simulink model "RC_top_ACU"  (R2018b)
settings: Solver=VariableStepAuto  StartTime=0.0  StopTime=500000.0  RelTol=1e-3
libraries: simulink x4
(part 1 of 3)
settings Model: Creator=user  LastModifiedBy=user

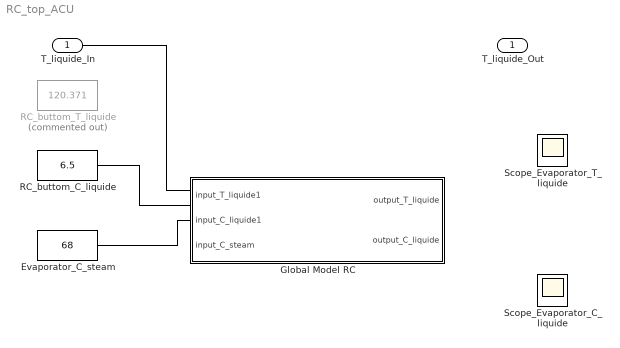
== system RC_top_ACU ==
  T_liquide_In : Inport
  Evaporator_C_steam : Constant  Value=68
  Global Model RC : Subsystem
  RC_buttom_C_liquide : Constant  Value=6.5
  RC_buttom_T_liquide : Constant  Commented=on  Value=120.371
  Scope_Evaporator_C_liquide : Scope
  Scope_Evaporator_T_liquide : Scope
  T_liquide_Out : Outport
  wires:
  ? -> T_liquide_Out/1, Scope_Evaporator_T_liquide/1
  ? -> Scope_Evaporator_C_liquide/1
  T_liquide_In/1 -> ?
  Evaporator_C_steam/1 -> ?
  RC_buttom_C_liquide/1 -> ?

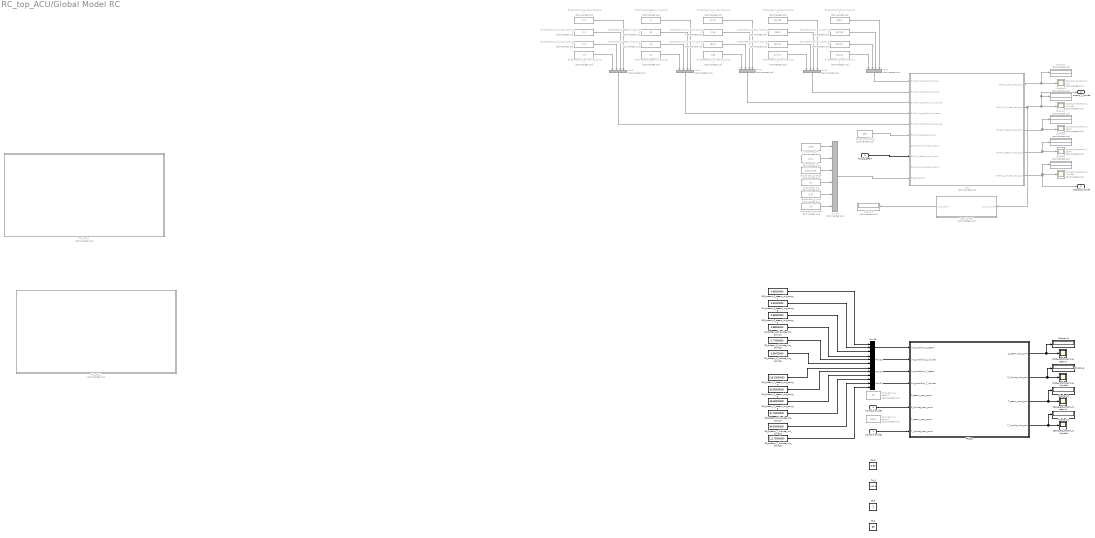
== system RC_top_ACU/Global Model RC ==
  input_T_liquide1 : Inport
  input_C_liquide1 : Inport  Port=2
  input_C_steam : Inport  Port=3
  ACU : Subsystem  Commented=on
  Cf_0 : Constant
  Cp_0 : Constant  Value=0.53
  Display{1..5,7} (6 alike) : Display  Commented=on
  Display{6,12..14} (4 alike) : Display
  Evaporator_C_liquide_init_point_1 : Constant  Commented=on  Value=2.2
  Evaporator_C_liquide_init_point_2 : Constant  Commented=on  Value=2.1
  Evaporator_C_liquide_init_point_3 : Constant  Commented=on  Value=2.0
  Evaporator_C_liquide_init_point_4 : Constant  Commented=on  Value=1.9
  Evaporator_C_steam_init_point_1 : Constant  Commented=on  Value=5
  Evaporator_C_steam_init_point_2 : Constant  Commented=on  Value=10
  Evaporator_C_steam_init_point_3 : Constant  Commented=on  Value=15
  Evaporator_C_steam_init_point_4 : Constant  Commented=on  Value=20
  Evaporator_Diameter : Constant  Commented=on  Value=5.5
  Evaporator_G_steam : Constant  Commented=on  Value=0.0017763
  Evaporator_P_0 : Constant  Commented=on  Value=0.1
  Evaporator_P_work : Constant  Commented=on  Value=0.06
  Evaporator_T_flue : Constant  Commented=on  Value=360
  Evaporator_T_flue_init_point_1 : Constant  Commented=on  Value=283.3
  Evaporator_T_flue_init_point_2 : Constant  Commented=on  Value=267.89
  Evaporator_T_flue_init_point_3 : Constant  Commented=on  Value=253.67
  Evaporator_T_flue_init_point_4 : Constant  Commented=on  Value=240.54
  Evaporator_T_liquide_init_point_1 : Constant  Commented=on  Value=137.5
  Evaporator_T_liquide_init_point_2 : Constant  Commented=on  Value=145
  Evaporator_T_liquide_init_point_3 : Constant  Commented=on  Value=152.5
  Evaporator_T_liquide_init_point_4 : Constant  Commented=on  Value=158
  Evaporator_T_side_init_point_1 : Constant  Commented=on  Value=164.48
  Evaporator_T_side_init_point_2 : Constant  Commented=on  Value=158.3
  Evaporator_T_side_init_point_3 : Constant  Commented=on  Value=152.41
  Evaporator_T_side_init_point_4 : Constant  Commented=on  Value=147.07
  Evaporator_Vm : Constant  Commented=on  Value=22.4
  Evaporator_dh : Constant  Commented=on  Value=1.375
  FULL_RC_1 : Subsystem  Commented=on
  FULL_RC_2 : Subsystem  Commented=on
  Local Control : Subsystem  Commented=on
  Mux10 : Mux  Commented=on  Inputs=6
  Mux{11..14} (4 alike) : Mux  Inputs=3
  Mux{5..9} (5 alike) : Mux  Commented=on
  RC_buttom_C_liquide_init_point_4 : Constant  Value=0.88825000
  RC_buttom_C_liquide_init_point_5 : Constant  Value=0.77650000
  RC_buttom_C_liquide_init_point_6 : Constant  Value=0.66475000
  RC_buttom_C_steam1 : Constant  Commented=on  Value=50
  RC_buttom_C_steam_init_point_4 : Constant  Value=0.68200000
  RC_buttom_C_steam_init_point_5 : Constant  Value=0.83400000
  RC_buttom_C_steam_init_point_6 : Constant  Value=0.98600000
  RC_buttom_T_liquide_init_point_4 : Constant  Value=57.25000000
  RC_buttom_T_liquide_init_point_5 : Constant  Value=84.50000000
  RC_buttom_T_liquide_init_point_6 : Constant  Value=111.75000000
  RC_buttom_T_steam1 : Constant  Commented=on  Value=150.4
  RC_buttom_T_steam_init_point_4 : Constant  Value=118.20000000
  RC_buttom_T_steam_init_point_5 : Constant  Value=93.90000000
  RC_buttom_T_steam_init_point_6 : Constant  Value=69.60000000
  RC_top : Subsystem
  Scope_Evaporator_C_liquide1 : Scope  Commented=on
  Scope_Evaporator_C_steam : Scope  Commented=on
  Scope_Evaporator_T_flue : Scope  Commented=on
  Scope_Evaporator_T_liquide1 : Scope  Commented=on
  Scope_Evaporator_T_steam : Scope  Commented=on
  Scope_RC_buttom_C_liquide1 : Scope
  Scope_RC_buttom_C_steam1 : Scope
  Scope_RC_buttom_T_liquide1 : Scope
  Scope_RC_buttom_T_steam1 : Scope
  Tf_0 : Constant  Value=30
  Tp_0 : Constant  Value=142.5
  output_T_liquide : Outport
  output_C_liquide : Outport  Port=2
  wires:
  RC_buttom_C_steam_init_point_6/1 -> Mux13/3
  RC_buttom_T_steam_init_point_6/1 -> Mux14/3
  RC_buttom_T_liquide_init_point_5/1 -> Mux12/2
  RC_buttom_C_steam_init_point_5/1 -> Mux13/2
  RC_buttom_C_liquide_init_point_5/1 -> Mux11/2
  RC_buttom_T_liquide_init_point_4/1 -> Mux12/1
  RC_top/1(C_steam_next_point) -> Display14/1, Scope_RC_buttom_C_steam1/1
  RC_buttom_C_liquide_init_point_4/1 -> Mux11/1
  Mux14/1 -> RC_top/3(init_condition_T_steam)
  input_C_liquide1/1 -> RC_top/6(C_liquide_prev_point)
  RC_top/2(C_liquide_next_point) -> Display6/1, Scope_RC_buttom_C_liquide1/1
  Mux12/1 -> RC_top/4(init_condition_T_liquide)
  RC_buttom_T_steam_init_point_5/1 -> Mux14/2
  Mux13/1 -> RC_top/1(init_condition_C_steam)
  input_T_liquide1/1 -> RC_top/8(T_liquide_prev_point)
  RC_buttom_T_liquide_init_point_6/1 -> Mux12/3
  RC_buttom_T_steam_init_point_4/1 -> Mux14/1
  RC_buttom_C_liquide_init_point_6/1 -> Mux11/3
  Mux11/1 -> RC_top/2(init_condition_C_liquide)
  RC_buttom_C_steam_init_point_4/1 -> Mux13/1
  RC_top/4(T_liquide_next_point) -> Display12/1, Scope_RC_buttom_T_liquide1/1
  RC_top/3(T_steam_next_point) -> Display13/1, Scope_RC_buttom_T_steam1/1
  Evaporator_T_liquide_init_point_3/1 -> Mux8/2
  Evaporator_T_side_init_point_4/1 -> Mux5/1
  Evaporator_T_side_init_point_2/1 -> Mux5/3
  Evaporator_C_steam_init_point_2/1 -> Mux6/3
  Evaporator_C_steam_init_point_3/1 -> Mux6/2
  Mux5/1 -> ACU/2(EVAP_init_condition_T_side)
  Evaporator_Vm/1 -> Mux10/2
  Mux7/1 -> ACU/1(EVAP_init_condition_T_flue)
  ACU/5(EVAP_C_liquide_next_point) -> Display7/1, Scope_Evaporator_C_liquide1/1, output_C_liquide/1
  ACU/1(EVAP_T_flue_next_point) -> Display2/1, Scope_Evaporator_T_flue/1
  Evaporator_C_steam_init_point_1/1 -> Mux6/4
  Evaporator_G_steam/1 -> Mux10/3
  Evaporator_T_liquide_init_point_1/1 -> Mux8/4
  ACU/4(EVAP_C_steam_next_point) -> Display4/1, Scope_Evaporator_C_steam/1
  Evaporator_C_liquide_init_point_3/1 -> Mux9/2
  Evaporator_P_work/1 -> Mux10/5
  Evaporator_T_flue_init_point_1/1 -> Mux7/4
  Evaporator_T_flue_init_point_4/1 -> Mux7/1
  Evaporator_T_liquide_init_point_4/1 -> Mux8/1
  Local Control/1(curr_T_flue) -> Display5/1
  Evaporator_C_liquide_init_point_2/1 -> Mux9/3
  Mux8/1 -> ACU/3(EVAP_init_condition_T_liquide)
  Evaporator_T_flue_init_point_2/1 -> Mux7/3
  Mux6/1 -> ACU/4(EVAP_init_condition_C_steam)
  Evaporator_P_0/1 -> Mux10/4
  Mux10/1 -> ACU/10(EVAP_params)
  Evaporator_T_flue_init_point_3/1 -> Mux7/2
  input_C_steam/1 -> ACU/8(EVAP_C_steam_prev_point)
  Evaporator_C_liquide_init_point_4/1 -> Mux9/1
  Evaporator_dh/1 -> Mux10/1
  Evaporator_T_side_init_point_3/1 -> Mux5/2
  ACU/3(EVAP_T_steam_next_point) -> Display1/1, Scope_Evaporator_T_steam/1
  Evaporator_Diameter/1 -> Mux10/6
  Mux9/1 -> ACU/5(EVAP_init_condition_C_liquide)
  Evaporator_C_steam_init_point_4/1 -> Mux6/1
  Evaporator_T_flue/1 -> ACU/6(EVAP_T_flue_prev_point)
  Evaporator_C_liquide_init_point_1/1 -> Mux9/4
  Evaporator_T_side_init_point_1/1 -> Mux5/4
  Evaporator_T_liquide_init_point_2/1 -> Mux8/3
  ACU/2(EVAP_T_liquide_next_point) -> output_T_liquide/1, Display3/1, Scope_Evaporator_T_liquide1/1, Local Control/1(curr_T_liquide)

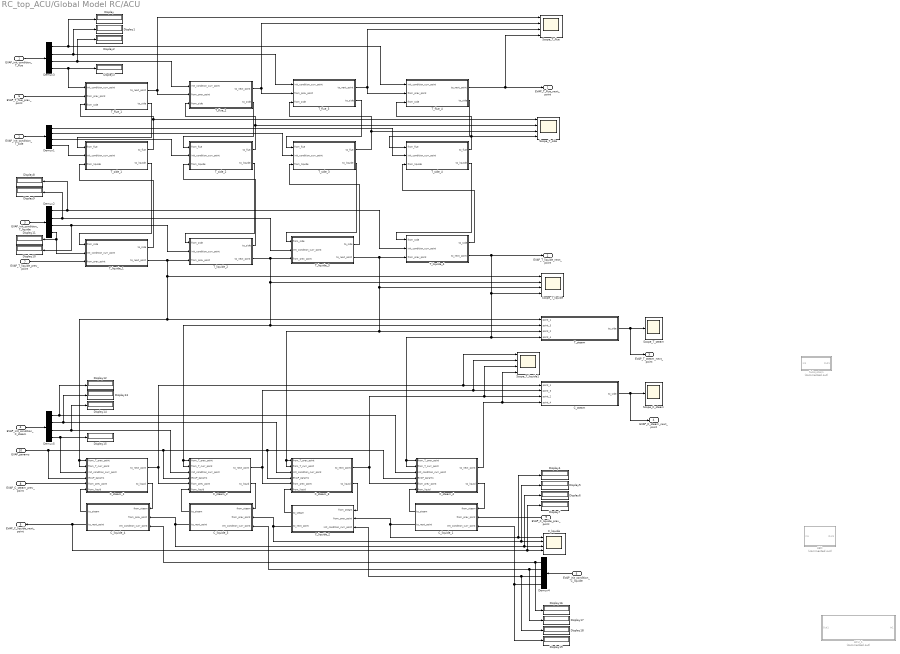
== system RC_top_ACU/Global Model RC/ACU ==
  EVAP_init_condition_T_flue : Inport
  EVAP_init_condition_T_side : Inport  Port=2
  EVAP_init_condition_T_liquide : Inport  Port=3
  EVAP_init_condition_C_steam : Inport  Port=4
  EVAP_init_condition_C_liquide : Inport  Port=5
  EVAP_T_flue_prev_point : Inport  Port=6
  EVAP_T_liquide_prev_point : Inport  Port=7
  EVAP_C_steam_prev_point : Inport  Port=8
  EVAP_C_liquide_prev_point : Inport  Port=9
  EVAP_params : Inport  Port=10
  "ACU_1 " : Subsystem  Commented=on
  C_liquide : Scope  NumInputPorts=4
  C_liquide_1 : Subsystem
  C_liquide_2 : Subsystem
  C_liquide_3 : Subsystem
  C_liquide_4 : Subsystem
  C_steam : Subsystem
  C_steam_1 : Subsystem
  C_steam_2 : Subsystem
  C_steam_3 : Subsystem
  C_steam_4 : Subsystem
  Demux{1..5} (5 alike) : Demux
  Display{,1..19} (20 alike) : Display
  Scope_C_steam : Scope
  Scope_T_flue : Scope  NumInputPorts=4
  Scope_T_liquide : Scope  NumInputPorts=4
  Scope_T_liquide1 : Scope  NumInputPorts=4
  Scope_T_side : Scope  NumInputPorts=4
  Scope_T_steam : Scope
  Subsystem : Subsystem  Commented=on
  T_flue_1 : Subsystem
  T_flue_2 : Subsystem
  T_flue_3 : Subsystem
  T_flue_4 : Subsystem
  T_liquide_1 : Subsystem
  T_liquide_2 : Subsystem
  T_liquide_3 : Subsystem
  T_liquide_4 : Subsystem
  T_side_1 : Subsystem
  T_side_2 : Subsystem
  T_side_3 : Subsystem
  T_side_4 : Subsystem
  T_steam : Subsystem
  АВО : Subsystem  Commented=on
  EVAP_T_flue_next_point : Outport
  EVAP_T_liquide_next_point : Outport  Port=2
  EVAP_T_steam_next_point : Outport  Port=3
  EVAP_C_steam_next_point : Outport  Port=4
  EVAP_C_liquide_next_point : Outport  Port=5
  wires:
  T_liquide_3/2(to_next_point) -> T_liquide_4/3(from_prev_point), C_steam_3/1(from_T_prev_point), C_steam_3/2(from_T_curr_point), T_steam/3(point_2), Scope_T_liquide/3
  EVAP_init_condition_T_liquide/1 -> Demux2/1
  Demux2/1 -> T_liquide_4/2(init_condition_curr_point), Display8/1
  EVAP_init_condition_T_side/1 -> Demux1/1
  T_liquide_4/2(to_next_point) -> Scope_T_liquide/4, C_steam_4/2(from_T_curr_point), C_steam_4/1(from_T_prev_point), T_steam/4(point_4), EVAP_T_liquide_next_point/1
  Demux2/2 -> T_liquide_3/2(init_condition_curr_point), Display9/1
  Demux2/4 -> T_liquide_1/2(init_condition_curr_point), Display11/1
  EVAP_init_condition_T_flue/1 -> Demux3/1
  T_flue_1/1(to_next_point) -> T_flue_2/2(from_prev_point), Scope_T_flue/1
  T_flue_2/1(to_next_point) -> T_flue_3/2(from_prev_point), Scope_T_flue/2
  T_flue_3/1(to_next_point) -> T_flue_4/2(from_prev_point), Scope_T_flue/3
  Demux3/1 -> T_flue_4/1(init_condition_curr_point), Display/1
  Demux3/2 -> T_flue_3/1(init_condition_curr_point), Display1/1
  Demux3/3 -> T_flue_2/1(init_condition_curr_point), Display2/1
  Demux3/4 -> T_flue_1/1(init_condition_curr_point), Display3/1
  T_flue_4/1(to_next_point) -> EVAP_T_flue_next_point/1, Scope_T_flue/4
  EVAP_T_flue_prev_point/1 -> T_flue_1/2(from_prev_point)
  T_steam/1(to_side) -> EVAP_T_steam_next_point/1, Scope_T_steam/1
  Demux5/2 -> C_steam_3/3(init_condition_curr_point), Display13/1
  C_liquide_2/2(to_next_point) -> C_liquide_3/2(from_prev_point), Display5/1, C_liquide/2
  C_steam_2/1(to_next_point) -> C_steam_3/5(from_prev_point), Scope_T_liquide1/2, C_steam/2(point_3)
  EVAP_init_condition_C_liquide/1 -> Demux4/1
  Demux5/3 -> C_steam_2/3(init_condition_curr_point), Display14/1
  C_steam_1/2(to_liquid) -> C_liquide_4/1(from_steam)
  Demux5/1 -> C_steam_4/3(init_condition_curr_point), Display12/1
  EVAP_init_condition_C_steam/1 -> Demux5/1
  EVAP_C_steam_prev_point/1 -> C_steam_1/5(from_prev_point)
  C_liquide_4/2(to_next_point) -> EVAP_C_liquide_next_point/1, Display7/1, C_liquide/4
  C_liquide_2/1(to_steam) -> C_steam_3/6(from_liquid)
  C_liquide_3/2(to_next_point) -> C_liquide_4/2(from_prev_point), Display6/1, C_liquide/3
  C_liquide_4/1(to_steam) -> C_steam_1/6(from_liquid)
  C_steam_3/1(to_next_point) -> C_steam_4/5(from_prev_point), Scope_T_liquide1/3, C_steam/3(point_2)
  EVAP_C_liquide_prev_point/1 -> C_liquide_1/2(from_prev_point)
  C_steam_4/2(to_liquid) -> C_liquide_1/1(from_steam)
  C_liquide_1/1(to_steam) -> C_steam_4/6(from_liquid)
  Demux5/4 -> C_steam_1/3(init_condition_curr_point), Display15/1
  C_liquide_1/2(to_next_point) -> C_liquide_2/2(from_prev_point), Display4/1, C_liquide/1
  Demux4/1 -> C_liquide_4/3(init_condition_curr_point), Display16/1
  Demux4/2 -> C_liquide_3/3(init_condition_curr_point), Display17/1
  Demux4/3 -> C_liquide_2/3(init_condition_curr_point), Display18/1
  Demux4/4 -> C_liquide_1/3(init_condition_curr_point), Display19/1
  C_steam/1(to_side) -> EVAP_C_steam_next_point/1, Scope_C_steam/1
  C_steam_1/1(to_next_point) -> C_steam_2/5(from_prev_point), Scope_T_liquide1/1, C_steam/1(point_1)
  C_steam_4/1(to_next_point) -> Scope_T_liquide1/4, C_steam/4(point_4)
  EVAP_params/1 -> C_steam_1/4(EVAP_params), C_steam_2/4(EVAP_params), C_steam_4/4(EVAP_params), C_steam_3/4(EVAP_params)
  C_liquide_3/1(to_steam) -> C_steam_2/6(from_liquid)
  C_steam_2/2(to_liquid) -> C_liquide_3/1(from_steam)
  EVAP_T_liquide_prev_point/1 -> T_liquide_1/3(from_prev_point)
  C_steam_3/2(to_liquid) -> C_liquide_2/1(from_steam)
  T_liquide_1/2(to_next_point) -> T_liquide_2/3(from_prev_point), Scope_T_liquide/1, T_steam/1(point_1), C_steam_1/1(from_T_prev_point), C_steam_1/2(from_T_curr_point)
  Demux2/3 -> T_liquide_2/2(init_condition_curr_point), Display10/1
  T_side_1/1(to_flue) -> Scope_T_side/1, T_flue_1/3(from_side)
  T_flue_1/2(to_side) -> T_side_1/1(from_flue)
  T_side_1/2(to_liquide) -> T_liquide_1/1(from_side)
  T_liquide_1/1(to_side) -> T_side_1/3(from_liquide)
  Demux1/4 -> T_side_1/2(init_condition_curr_point)
  T_side_2/1(to_flue) -> T_flue_2/3(from_side), Scope_T_side/2
  T_flue_2/2(to_side) -> T_side_2/1(from_flue)
  T_side_3/1(to_flue) -> T_flue_3/3(from_side), Scope_T_side/3
  T_flue_3/2(to_side) -> T_side_3/1(from_flue)
  T_side_4/1(to_flue) -> T_flue_4/3(from_side), Scope_T_side/4
  T_flue_4/2(to_side) -> T_side_4/1(from_flue)
  T_liquide_2/1(to_side) -> T_side_2/3(from_liquide)
  T_side_2/2(to_liquide) -> T_liquide_2/1(from_side)
  T_side_3/2(to_liquide) -> T_liquide_3/1(from_side)
  T_liquide_3/1(to_side) -> T_side_3/3(from_liquide)
  T_side_4/2(to_liquide) -> T_liquide_4/1(from_side)
  T_liquide_4/1(to_side) -> T_side_4/3(from_liquide)
  Demux1/3 -> T_side_2/2(init_condition_curr_point)
  Demux1/2 -> T_side_3/2(init_condition_curr_point)
  Demux1/1 -> T_side_4/2(init_condition_curr_point)
  T_liquide_2/2(to_next_point) -> T_liquide_3/3(from_prev_point), C_steam_2/2(from_T_curr_point), C_steam_2/1(from_T_prev_point), T_steam/2(point_3), Scope_T_liquide/2

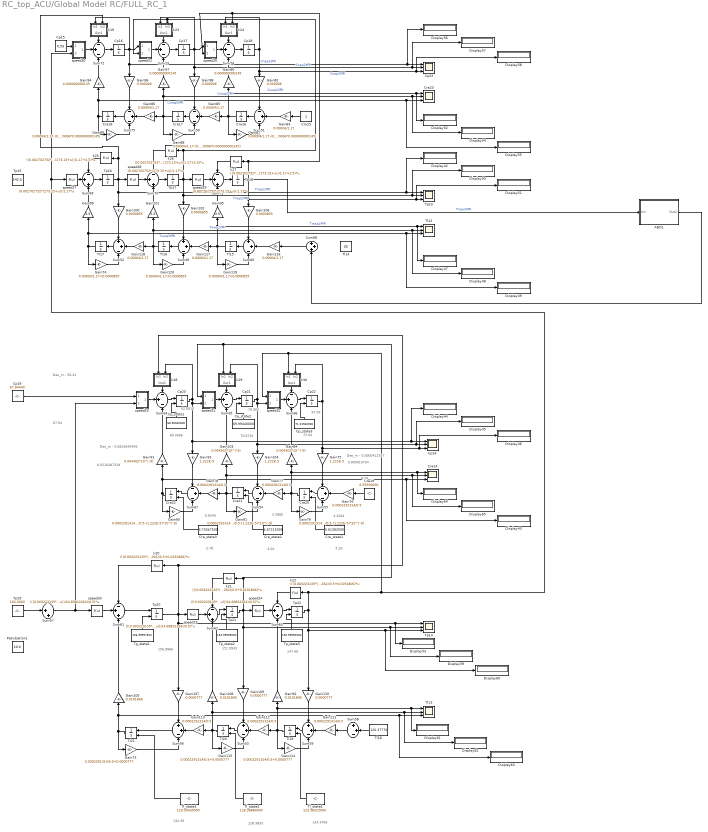
== system RC_top_ACU/Global Model RC/FULL_RC_1 ==
  note: 4.2264
  note: 69.3066
  note: 72.04
  note: 156.9966
  note: 124.3766
  note: 0.000010734
  note: 4.24
  note: Des_m - 0.0000412357
  note: 67.94
  note: Des_m - 50.41
  note: 4.02
  note: 147.99
  note: Des_m - 0.0815645409
  note: 0.0216487318
  note: 70.6733
  note: 2.3980
  note: 2.78
  note: 5.26
  note: 78.085
  note: 97.09
  note: 62.8910
  note: 0.9249
  note: 128.3833
  note: 151.9933
  note: 132.39
  Cp14 : Scope  NumInputPorts=3
  Cp15 : Constant  Value=0.53
  Cp16 : Integrator  InitialCondition=0.665
  Cp17 : Integrator  InitialCondition=0.803
  Cp18 : Integrator  InitialCondition=0.986
  Cp19 : Constant  Value=67.94440
  Cp20 : Integrator  InitialConditionSource=external  InitialCondition=69.3066
  Cp21 : Integrator  InitialConditionSource=external  InitialCondition=70.6733
  Cp22 : Integrator  InitialConditionSource=external  InitialCondition=72.04
  Cp23 : Scope  NumInputPorts=3
  Cp_state1 : Constant  Value=68.96940000
  Cp_state2 : Constant  Value=69.99440000
  Cp_state3 : Constant  Value=71.01940000
  Cra14 : Scope  NumInputPorts=3
  Cra15 : Constant
  Cra16 : Integrator  InitialCondition=0.827
  Cra17 : Integrator  InitialCondition=0.6862
  Cra18 : Integrator  InitialCondition=0.5696
  Cra19 : Constant  Value=6.55550000
  Cra20 : Integrator  InitialConditionSource=external  InitialCondition=5.26
  Cra21 : Integrator  InitialConditionSource=external  InitialCondition=4.02
  Cra22 : Integrator  InitialConditionSource=external  InitialCondition=2.78
  Cra23 : Scope  NumInputPorts=3
  Cra_state1 : Constant  Value=5.61382500
  Cra_state2 : Constant  Value=4.67215000
  Cra_state3 : Constant  Value=3.73047500
  Display{42..65} (24 alike) : Display
  Gain100 : Gain  Gain=0.0000855
  Gain101 : Gain  Gain=2.5
  Gain102 : Gain  Gain=0.0000855
  Gain103 : Gain  Gain=0.004302*10^(-9)
  Gain104 : Gain  Gain=1.222E-5
  Gain105 : Gain  Gain=0.0191806
  Gain106 : Gain  Gain=0.0000855
  Gain107 : Gain  Gain=0.0000777
  Gain108 : Gain  Gain=0.0191806
  Gain109 : Gain  Gain=0.0000777
  Gain110 : Gain  Gain=0.0000777
  Gain{76..78,111..113} (6 alike) : Gain  Gain=0.0002291314/0.5
  Gain114 : Gain  Gain=0.0002291314/0.5+0.0000777
  Gain115 : Gain  Gain=0.0002291314/0.5+0.0000777
  Gain{83,85..86,116..118} (6 alike) : Gain  Gain=0.00004/1.17
  Gain119 : Gain  Gain=0.00004/1.17+0.0000855
  Gain120 : Gain  Gain=0.00004/1.17+0.0000855
  Gain73 : Gain  Gain=0.0002291314/0.5+0.0000777
  Gain74 : Gain  Gain=0.00004/1.17+0.0000855
  Gain75 : Gain  Gain=1.222E-5
  Gain79 : Gain  Gain=0.0002291314/0.5-(1.222E-5)*10^(-9)
  Gain80 : Gain  Gain=0.000000000145
  Gain81 : Gain  Gain=0.0002291314/0.5-(1.222E-5)*10^(-9)
  Gain82 : Gain  Gain=0.000006
  Gain84 : Gain  Gain=0.004302*10^(-9)
  Gain87 : Gain  Gain=0.00004/1.17-(0.000006*0.000000000145)
  Gain88 : Gain  Gain=0.00004/1.17-(0.000006*0.000000000145)
  Gain89 : Gain  Gain=0.00004/1.17-(0.000006*0.000000000145)
  Gain90 : Gain  Gain=0.0002291314/0.5-(1.222E-5)*10^(-9)
  Gain91 : Gain  Gain=0.004302*10^(-9)
  Gain92 : Gain  Gain=0.0191806
  Gain93 : Gain  Gain=1.222E-5
  Gain94 : Gain  Gain=0.000000000145
  Gain95 : Gain  Gain=2.5
  Gain96 : Gain  Gain=0.000006
  Gain97 : Gain  Gain=0.000000000145
  Gain98 : Gain  Gain=0.000006
  Gain99 : Gain  Gain=2.5
  Petrubation1 : Constant  Value=10.0
  Sum{49,52..53,56,58..60} (7 alike) : Sum  Inputs=++-
  Sum{50..51,54..55,64..67,72..75} (12 alike) : Sum  Inputs=-+-
  Sum57 : Sum  Inputs=|++
  Sum{61..63,69..71} (6 alike) : Sum  Inputs=-++
  Sum68 : Sum  Inputs=+++
  Tl13 : Scope  NumInputPorts=3
  Tl14 : Constant  Value=30
  Tl15 : Integrator  InitialCondition=58.28
  Tl16 : Integrator  InitialCondition=86.23
  Tl17 : Integrator  InitialCondition=111.75
  Tl18 : Constant  Value=120.37770
  Tl19 : Integrator  InitialConditionSource=external  InitialCondition=124.3766
  Tl20 : Integrator  InitialConditionSource=external  InitialCondition=128.3833
  Tl21 : Integrator  InitialConditionSource=external  InitialCondition=132.39
  Tl22 : Scope  NumInputPorts=3
  "Tl_state1 " : Constant  Value=123.38325000
  Tl_state2 : Constant  Value=126.38880000
  Tl_state3 : Constant  Value=129.39435000
  Tp14 : Scope  NumInputPorts=3
  Tp15 : Constant  Value=142.5
  Tp16 : Integrator  InitialCondition=121.956
  Tp17 : Integrator  InitialCondition=97.4
  Tp18 : Integrator  InitialCondition=69.6  IgnoreLimit=on
  Tp19 : Constant  Value=160.0000
  Tp20 : Integrator  InitialConditionSource=external  InitialCondition=156.9966
  Tp21 : Integrator  InitialConditionSource=external  InitialCondition=151.9933
  Tp22 : Integrator  InitialConditionSource=external  InitialCondition=147.99  IgnoreLimit=on
  Tp23 : Scope  NumInputPorts=3
  Tp_state1 : Constant  Value=156.99997500
  Tp_state2 : Constant  Value=153.99995000
  Tp_state3 : Constant  Value=150.99992500
  k19 : Subsystem
  k20 : Fcn  Expr=(((0.003223135*(273+u))/24.69822264)/0.5+0.0191806)*u
  k21 : Fcn  Expr=(((0.003223135*(273+u))/24.69822264)/0.5+0.0191806)*u
  k22 : Fcn  Expr=(((0.003223135*(273+u))/24.69822264)/0.5+0.0191806)*u
  k23 : Subsystem
  k24 : Subsystem
  k25 : Fcn  Expr=((0.002702752*(273.15+u))/1.17+2.5)*u
  k26 : Fcn  Expr=((0.002702752*(273.15+u))/1.17+2.5)*u
  k27 : Fcn  Expr=((0.002702752*(273.15+u))/1.17+2.5)*u
  k28 : Subsystem
  k29 : Subsystem
  k30 : Subsystem
  speed22 : Subsystem
  speed23 : Fcn  Expr=(((0.003223135*(273+u))/24.69822264)/0.5)*u
  speed24 : Fcn  Expr=(((0.003223135*(273+u))/24.69822264)/0.5)*u
  speed25 : Subsystem
  speed26 : Subsystem
  speed27 : Fcn  Expr=(0.002702752*(273.15+u))/1.17*u
  speed28 : Fcn  Expr=(0.002702752*(273.15+u))/1.17*u
  speed29 : Fcn  Expr=(0.002702752*(273.15+u))/1.17*u
  speed30 : Subsystem
  speed31 : Subsystem
  speed32 : Subsystem
  speed33 : Fcn  Expr=(((0.003223135*(273+u))/24.69822264)/0.5)*u
  АВО1 : Subsystem
  wires:
  k30/1(Out1) -> Sum66/1
  Tl19/1 -> Gain114/1, Gain112/1, Gain92/1, Display61/1, Tl13/1
  speed25/1(Out1) -> Sum64/2
  Tp_state1/1 -> Tp20/2
  Gain109/1 -> Sum53/1
  Gain113/1 -> Sum56/2
  speed22/1(Out1) -> Sum73/2
  Cp20/1 -> speed31/2(In2), Gain93/1, Cp14/1, Display44/1, k28/2(In2)
  Tl21/1 -> Gain73/1, Gain105/1, Display63/1, Tl13/3
  Cp15/1 -> speed30/1(In1)
  Sum63/1 -> Tp22/1
  Cp16/1 -> Cp23/1, Display56/1, Gain96/1, k19/1(In1), speed22/1(In1)  "Cпар1УРК"
  Tp16/1 -> Display42/1, Tp23/1, Gain100/1, k25/1, k19/2(In2), speed28/1  "Tпар1УРК"
  speed26/1(Out1) -> Sum74/2
  Gain89/1 -> Sum75/3
  speed27/1 -> Sum69/2
  Sum49/1 -> Tl16/1
  Sum56/1 -> Tl21/1
  k27/1 -> Sum71/1
  Gain116/1 -> Sum60/2
  Gain81/1 -> Sum54/3
  k26/1 -> Sum70/1
  speed31/1(Out1) -> Sum65/2
  Gain99/1 -> Sum69/3
  Gain94/1 -> Sum72/3
  Sum73/1 -> Cp17/1
  Gain82/1 -> Sum51/1
  Sum74/1 -> Cp18/1
  Sum69/1 -> Tp16/1
  Cra19/1 -> Gain76/1
  k20/1 -> Sum61/1
  Gain97/1 -> Sum73/3
  Tp18/1 -> АВО1/1(In1), Display51/1, Tp23/3, Gain106/1, k27/1, k24/2(In2), speed26/2(In2)  "Tпар3УРК"
  Gain91/1 -> Sum64/3
  speed23/1 -> Sum62/2
  Gain80/1 -> Sum74/3
  "Tl_state1 "/1 -> Tl19/2
  Tp20/1 -> Gain107/1, Display53/1, Tp14/1, k20/1, k28/1(In1), speed23/1
  Gain95/1 -> Sum71/3
  Sum50/1 -> Cra17/1
  Gain98/1 -> Sum50/1
  k19/1(Out1) -> Sum72/1
  Gain106/1 -> Sum60/1
  Tp21/1 -> Gain109/1, Display59/1, Tp14/2, k21/1, speed31/1(In1), k29/1(In1), speed24/1
  Tp_state3/1 -> Tp22/2
  k21/1 -> Sum62/1
  Sum75/1 -> Cra18/1
  speed30/1(Out1) -> Sum72/2
  Sum72/1 -> Cp16/1
  Sum52/1 -> Tl17/1
  Cp_state3/1 -> Cp22/2
  Gain120/1 -> Sum49/3
  Gain79/1 -> Sum55/3
  Sum70/1 -> Tp17/1
  Tl15/1 -> Gain119/1, Gain117/1, Display47/1, Tl22/1, Gain95/1  "Tжид1УРК"
  Gain85/1 -> Sum50/2
  Tl18/1 -> Sum58/2
  Cp17/1 -> Display57/1, Cp23/2, Gain98/1, speed26/1(In1), k23/1(In1)  "Cпар2УРК"
  Tl_state3/1 -> Tl21/2
  Gain100/1 -> Sum52/1
  Tl16/1 -> Gain120/1, Gain118/1, Display48/1, Tl22/2, Gain101/1  "Tжид2УРК"
  Cra17/1 -> Gain88/1, Gain86/1, Display54/1, Cra23/2, Gain97/1  "Cжид2УРК"
  Gain104/1 -> Sum54/1
  Sum57/1 -> speed33/1, speed25/2(In2)
  Gain78/1 -> Sum67/2
  Cp22/1 -> k30/2(In2), Gain75/1, Display46/1, Cp14/3
  Gain84/1 -> Sum66/3
  Gain117/1 -> Sum49/2
  Sum65/1 -> Cp21/1
  Gain118/1 -> Sum52/2
  Gain87/1 -> Sum51/3
  Cra20/1 -> Gain79/1, Gain77/1, Gain84/1, Display64/1, Cra14/1
  Sum61/1 -> Tp20/1
  Sum62/1 -> Tp21/1
  Gain101/1 -> Sum70/3
  Gain86/1 -> Sum75/2
  Sum67/1 -> Cra22/1
  Gain75/1 -> Sum55/1
  speed28/1 -> Sum70/2
  Sum66/1 -> Cp22/1
  Sum58/1 -> Gain111/1
  Sum71/1 -> Tp18/1
  Gain111/1 -> Sum59/2
  speed29/1 -> Sum71/2
  Cra18/1 -> Gain89/1, Display55/1, Cra23/3, Gain94/1  "Cжид3УРК"
  k23/1(Out1) -> Sum73/1
  Gain110/1 -> Sum59/1
  Gain83/1 -> Sum51/2
  Sum55/1 -> Cra20/1
  k24/1(Out1) -> Sum74/1
  Gain119/1 -> Sum60/3
  Cra16/1 -> Gain87/1, Gain85/1, Display52/1, Cra23/1, Gain80/1  "Cжид1УРК"
  Gain114/1 -> Sum59/3
  Sum51/1 -> Cra16/1
  Gain90/1 -> Sum67/3
  k28/1(Out1) -> Sum64/1
  Gain88/1 -> Sum50/3
  Tl20/1 -> Gain115/1, Gain113/1, Gain108/1, Display62/1, Tl13/2
  Cra_state1/1 -> Cra20/2
  Tp22/1 -> Gain110/1, Display60/1, Tp14/3, k22/1, k30/1(In1), speed32/1(In1), speed30/2(In2), speed27/1
  Gain92/1 -> Sum63/3
  Cp_state2/1 -> Cp21/2
  Tp19/1 -> Sum57/1
  k25/1 -> Sum69/1
  Sum59/1 -> Tl19/1
  k22/1 -> Sum63/1
  speed24/1 -> Sum63/2
  Cp_state1/1 -> Cp20/2
  Gain105/1 -> Sum61/3
  Gain77/1 -> Sum54/2
  speed33/1 -> Sum61/2
  Gain112/1 -> Sum53/2
  k29/1(Out1) -> Sum65/1
  Cra15/1 -> Gain83/1
  Tp_state2/1 -> Tp21/2
  Gain93/1 -> Sum67/1
  Gain74/1 -> Sum52/3
  Tp17/1 -> Display50/1, Tp23/2, Gain102/1, k26/1, speed22/2(In2), k23/2(In2), speed29/1  "Tпар2УРК"
  Cra22/1 -> Gain90/1, Gain91/1, Display43/1, Cra14/3
  Sum64/1 -> Cp20/1
  Cra_state2/1 -> Cra21/2
  Cp19/1 -> speed25/1(In1)
  АВО1/1(Out1) -> Sum68/3
  Sum53/1 -> Tl20/1
  Gain115/1 -> Sum53/3
  Gain73/1 -> Sum56/3
  Tl_state2/1 -> Tl20/2
  Sum60/1 -> Tl15/1
  Gain76/1 -> Sum55/2
  Gain103/1 -> Sum65/3
  Cp21/1 -> speed32/2(In2), Gain104/1, Display45/1, Cp14/2, k29/2(In2)
  Cra_state3/1 -> Cra22/2
  Sum54/1 -> Cra21/1
  Gain96/1 -> Sum75/1
  Gain102/1 -> Sum49/1
  Cp18/1 -> Display58/1, Cp23/3, Gain82/1, k24/1(In1)  "Cпар3УРК"
  Gain108/1 -> Sum62/3
  Gain107/1 -> Sum56/1
  Cra21/1 -> Gain81/1, Gain78/1, Gain103/1, Display65/1, Cra14/2
  speed32/1(Out1) -> Sum66/2
  Tl17/1 -> Gain74/1, Display49/1, Tl22/3, Gain99/1  "Tжид3УРК"
  Sum68/1 -> Gain116/1

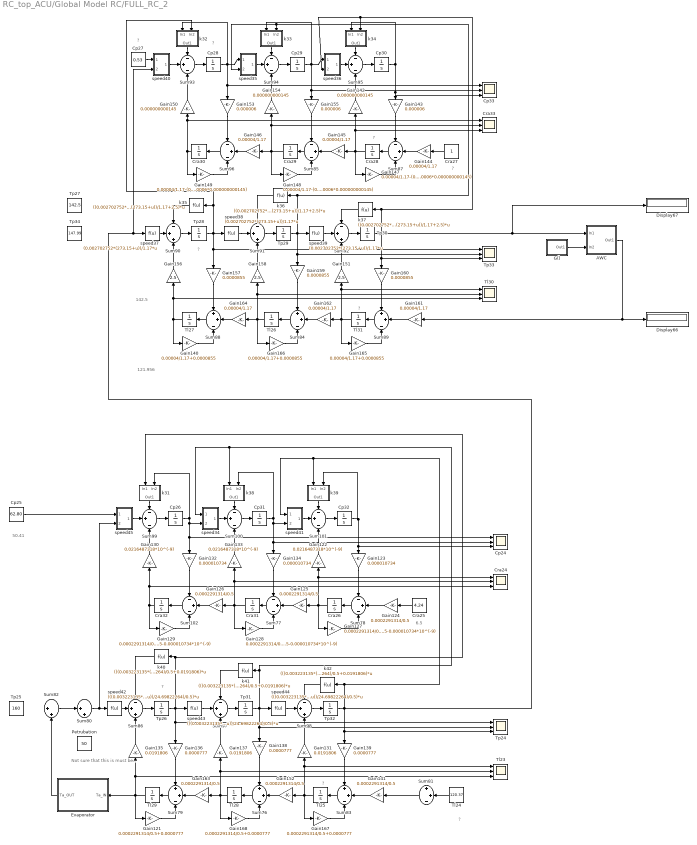
== system RC_top_ACU/Global Model RC/FULL_RC_2 ==
  note: ?
  note: Not sure that
      | this is must be..
  note: ?
  note: ?
  note: 142.5
  note: 50.41
  note: 6.5
  note: ?
  note: ?
  note: ?
  note: ?
  note: 121.956
  note: ?
  note: ?
  AWC : Subsystem
  Cp24 : Scope  NumInputPorts=3
  Cp25 : Constant  Value=62.80
  Cp26 : Integrator  InitialCondition=62.80
  Cp27 : Constant  Value=0.53
  Cp28 : Integrator  InitialCondition=0.665
  Cp29 : Integrator  InitialCondition=0.803
  Cp30 : Integrator  InitialCondition=0.986
  Cp31 : Integrator  InitialCondition=77.79
  Cp32 : Integrator  InitialCondition=96.56
  Cp33 : Scope  NumInputPorts=3
  Cra24 : Scope  NumInputPorts=3
  Cra25 : Constant  Value=4.24
  Cra26 : Integrator  InitialCondition=4.24
  Cra27 : Constant
  Cra28 : Integrator  InitialCondition=0.827
  Cra29 : Integrator  InitialCondition=0.6862
  Cra30 : Integrator  InitialCondition=0.5696
  Cra31 : Integrator  InitialCondition=2.42
  Cra32 : Integrator  InitialCondition=0.95
  Cra33 : Scope  NumInputPorts=3
  Display66 : Display
  Display67 : Display
  Evaporator : Subsystem
  G() : Subsystem
  Gain121 : Gain  Gain=0.0002291314/0.5+0.0000777
  Gain122 : Gain  Gain=0.0216487318*10^(-9)
  Gain123 : Gain  Gain=0.000010734
  Gain{124..126,141,152,163} (6 alike) : Gain  Gain=0.0002291314/0.5
  Gain127 : Gain  Gain=0.0002291314/0.5-0.000010734*10^(-9)
  Gain128 : Gain  Gain=0.0002291314/0.5-0.000010734*10^(-9)
  Gain129 : Gain  Gain=0.0002291314/0.5-0.000010734*10^(-9)
  Gain130 : Gain  Gain=0.0216487318*10^(-9)
  Gain131 : Gain  Gain=0.0191806
  Gain132 : Gain  Gain=0.000010734
  Gain133 : Gain  Gain=0.0216487318*10^(-9)
  Gain134 : Gain  Gain=0.000010734
  Gain135 : Gain  Gain=0.0191806
  Gain136 : Gain  Gain=0.0000777
  Gain137 : Gain  Gain=0.0191806
  Gain138 : Gain  Gain=0.0000777
  Gain139 : Gain  Gain=0.0000777
  Gain140 : Gain  Gain=0.00004/1.17+0.0000855
  Gain142 : Gain  Gain=0.000000000145
  Gain143 : Gain  Gain=0.000006
  Gain{144..146,161..162,164} (6 alike) : Gain  Gain=0.00004/1.17
  Gain147 : Gain  Gain=0.00004/1.17-(0.000006*0.000000000145)
  Gain148 : Gain  Gain=0.00004/1.17-(0.000006*0.000000000145)
  Gain149 : Gain  Gain=0.00004/1.17-(0.000006*0.000000000145)
  Gain150 : Gain  Gain=0.000000000145
  Gain151 : Gain  Gain=2.5
  Gain153 : Gain  Gain=0.000006
  Gain154 : Gain  Gain=0.000000000145
  Gain155 : Gain  Gain=0.000006
  Gain156 : Gain  Gain=2.5
  Gain157 : Gain  Gain=0.0000855
  Gain158 : Gain  Gain=2.5
  Gain159 : Gain  Gain=0.0000855
  Gain160 : Gain  Gain=0.0000855
  Gain165 : Gain  Gain=0.00004/1.17+0.0000855
  Gain166 : Gain  Gain=0.00004/1.17+0.0000855
  Gain167 : Gain  Gain=0.0002291314/0.5+0.0000777
  Gain168 : Gain  Gain=0.0002291314/0.5+0.0000777
  Petrubation : Constant  Value=50
  Sum{77..78,85,87,93..96,99..102} (12 alike) : Sum  Inputs=-+-
  Sum{76,79,81,83..84,88..89} (7 alike) : Sum  Inputs=++-
  Sum80 : Sum  Inputs=|++
  Sum82 : Sum  Inputs=|++
  Sum{86,90..92,97..98} (6 alike) : Sum  Inputs=-++
  Tl23 : Scope  NumInputPorts=3
  Tl24 : Constant  Value=120.37
  Tl25 : Integrator  InitialCondition=120.37
  Tl26 : Integrator  InitialCondition=86.23
  Tl27 : Integrator  InitialCondition=111.75
  Tl28 : Integrator  InitialCondition=124.37
  Tl29 : Integrator  InitialCondition=128.38
  Tl30 : Scope  NumInputPorts=3
  Tl31 : Integrator  InitialCondition=58.28
  Tp24 : Scope  NumInputPorts=3
  Tp25 : Constant  Value=160
  Tp26 : Integrator  InitialCondition=160
  Tp27 : Constant  Value=142.5
  Tp28 : Integrator  InitialCondition=121.956
  Tp29 : Integrator  InitialCondition=97.4
  Tp30 : Integrator  InitialCondition=69.6  IgnoreLimit=on
  Tp31 : Integrator  InitialCondition=157.34
  Tp32 : Integrator  InitialCondition=153.75  IgnoreLimit=on
  Tp33 : Scope  NumInputPorts=3
  Tp34 : Constant  Value=147.99
  k31 : Subsystem
  k32 : Subsystem
  k33 : Subsystem
  k34 : Subsystem
  k35 : Fcn  Expr=((0.002702752*(273.15+u))/1.17+2.5)*u
  k36 : Fcn  Expr=((0.002702752*(273.15+u))/1.17+2.5)*u
  k37 : Fcn  Expr=((0.002702752*(273.15+u))/1.17+2.5)*u
  k38 : Subsystem
  k39 : Subsystem
  k40 : Fcn  Expr=(((0.003223135*(273+u))/24.69822264)/0.5+0.0191806)*u
  k41 : Fcn  Expr=(((0.003223135*(273+u))/24.69822264)/0.5+0.0191806)*u
  k42 : Fcn  Expr=(((0.003223135*(273+u))/24.69822264)/0.5+0.0191806)*u
  speed34 : Subsystem
  speed35 : Subsystem
  speed36 : Subsystem
  speed37 : Fcn  Expr=(0.002702752*(273.15+u))/1.17*u
  speed38 : Fcn  Expr=(0.002702752*(273.15+u))/1.17*u
  speed39 : Fcn  Expr=(0.002702752*(273.15+u))/1.17*u
  speed40 : Subsystem
  speed41 : Subsystem
  speed42 : Fcn  Expr=(((0.003223135*(273+u))/24.69822264)/0.5)*u
  speed43 : Fcn  Expr=(((0.003223135*(273+u))/24.69822264)/0.5)*u
  speed44 : Fcn  Expr=(((0.003223135*(273+u))/24.69822264)/0.5)*u
  speed45 : Subsystem
  wires:
  Gain144/1 -> Sum87/2
  Sum85/1 -> Cra29/1
  Cra28/1 -> Gain147/1, Gain145/1, Cra33/3, Gain142/1
  Gain153/1 -> Sum96/1
  Cra30/1 -> Gain149/1, Cra33/1, Gain150/1
  Cp28/1 -> Cp33/1, Gain153/1, speed35/1(In1), k32/1(In1)
  Cra25/1 -> Gain124/1
  Cra31/1 -> Gain128/1, Gain126/1, Gain133/1, Cra24/2
  Cp32/1 -> k39/2(In2), Gain123/1, Cp24/3
  speed39/1 -> Sum92/2
  Gain146/1 -> Sum96/2
  k35/1 -> Sum90/1
  Sum97/1 -> Tp31/1
  Gain123/1 -> Sum78/1
  speed43/1 -> Sum97/2
  Sum96/1 -> Cra30/1
  Gain142/1 -> Sum95/3
  Tp32/1 -> Gain139/1, Tp24/3, speed40/2(In2), speed37/1, k42/1, k39/1(In1), speed41/1(In1)
  Tp31/1 -> Gain138/1, Tp24/2, k41/1, speed34/1(In1), k38/1(In1), speed44/1
  Cra27/1 -> Gain144/1
  Tp28/1 -> Gain157/1, Tp33/1, k35/1, k32/2(In2), speed38/1
  Sum81/1 -> Gain141/1
  Gain156/1 -> Sum90/3
  Gain151/1 -> Sum92/3
  Gain162/1 -> Sum84/2
  Gain155/1 -> Sum85/1
  Sum91/1 -> Tp29/1
  Tp29/1 -> Gain159/1, Tp33/2, k36/1, speed35/2(In2), k33/2(In2), speed39/1
  Tl31/1 -> Gain165/1, Gain162/1, Tl30/1, Gain151/1
  speed38/1 -> Sum91/2
  Cra32/1 -> Gain129/1, Gain130/1, Cra24/3
  Sum98/1 -> Tp32/1
  Gain163/1 -> Sum79/2
  Tl25/1 -> Gain167/1, Gain152/1, Gain131/1, Tl23/1
  k31/1(Out1) -> Sum99/1
  Sum78/1 -> Cra26/1
  speed41/1(Out1) -> Sum101/2
  Gain167/1 -> Sum83/3
  Gain150/1 -> Sum93/3
  Gain158/1 -> Sum91/3
  Cp29/1 -> Cp33/2, Gain155/1, speed36/1(In1), k33/1(In1)
  Sum94/1 -> Cp29/1
  k38/1(Out1) -> Sum100/1
  k40/1 -> Sum86/1
  Tl28/1 -> Gain168/1, Gain163/1, Gain137/1, Tl23/2
  Sum92/1 -> Tp30/1
  Gain154/1 -> Sum94/3
  Sum84/1 -> Tl26/1
  Gain121/1 -> Sum79/3
  k41/1 -> Sum97/1
  speed35/1(Out1) -> Sum94/2
  Gain131/1 -> Sum98/3
  Gain138/1 -> Sum76/1
  Gain141/1 -> Sum83/2
  Sum90/1 -> Tp28/1
  Gain157/1 -> Sum88/1
  Gain159/1 -> Sum84/1
  Gain136/1 -> Sum79/1
  Sum82/1 -> Sum80/1
  Gain128/1 -> Sum77/3
  Gain140/1 -> Sum88/3
  speed37/1 -> Sum90/2
  Sum99/1 -> Cp26/1
  k42/1 -> Sum98/1
  Sum80/1 -> speed45/2(In2), speed42/1
  Tp26/1 -> Gain136/1, Tp24/1, k40/1, k31/1(In1), speed43/1
  Sum89/1 -> Tl31/1
  Gain149/1 -> Sum96/3
  Gain148/1 -> Sum85/3
  k34/1(Out1) -> Sum95/1
  Cra29/1 -> Gain148/1, Gain146/1, Cra33/2, Gain154/1
  Tp30/1 -> AWC/1(In1), Display67/1, Gain160/1, Tp33/3, k37/1, k34/2(In2), speed36/2(In2)
  Sum93/1 -> Cp28/1
  Gain134/1 -> Sum77/1
  Gain127/1 -> Sum78/3
  Gain129/1 -> Sum102/3
  Gain161/1 -> Sum89/2
  speed42/1 -> Sum86/2
  Sum86/1 -> Tp26/1
  Cp26/1 -> speed34/2(In2), Gain132/1, Cp24/1, k31/2(In2)
  speed36/1(Out1) -> Sum95/2
  AWC/1(Out1) -> Display66/1, Gain161/1
  speed44/1 -> Sum98/2
  Sum102/1 -> Cra32/1
  Gain124/1 -> Sum78/2
  speed45/1(Out1) -> Sum99/2
  Sum77/1 -> Cra31/1
  Sum76/1 -> Tl28/1
  Tl26/1 -> Gain166/1, Gain164/1, Tl30/2, Gain158/1
  Gain135/1 -> Sum86/3
  Sum87/1 -> Cra28/1
  k36/1 -> Sum91/1
  speed34/1(Out1) -> Sum100/2
  Gain122/1 -> Sum101/3
  Evaporator/1(Ta_OUT) -> Sum82/2
  Sum88/1 -> Tl27/1
  speed40/1(Out1) -> Sum93/2
  Gain166/1 -> Sum84/3
  Gain145/1 -> Sum85/2
  Gain147/1 -> Sum87/3
  Gain152/1 -> Sum76/2
  Gain165/1 -> Sum89/3
  Cp25/1 -> speed45/1(In1)
  Cra26/1 -> Gain127/1, Gain125/1, Gain122/1, Cra24/1
  Gain143/1 -> Sum87/1
  Cp27/1 -> speed40/1(In1)
  Gain125/1 -> Sum77/2
  Gain168/1 -> Sum76/3
  Tl24/1 -> Sum81/2
  k37/1 -> Sum92/1
  Gain164/1 -> Sum88/2
  Sum79/1 -> Tl29/1
  k33/1(Out1) -> Sum94/1
  Gain130/1 -> Sum99/3
  Gain132/1 -> Sum102/1
  Gain126/1 -> Sum102/2
  Sum101/1 -> Cp32/1
  Cp31/1 -> speed41/2(In2), Gain134/1, Cp24/2, k38/2(In2)
  Cp30/1 -> Cp33/3, Gain143/1, k34/1(In1)
  Gain137/1 -> Sum97/3
  Tl29/1 -> Evaporator/1(Ta_IN), Gain121/1, Gain135/1, Tl23/3
  Gain133/1 -> Sum100/3
  k32/1(Out1) -> Sum93/1
  Gain160/1 -> Sum89/1
  Sum83/1 -> Tl25/1
  Gain139/1 -> Sum83/1
  k39/1(Out1) -> Sum101/1
  G()/1(Out1) -> AWC/2(In2)
  Tl27/1 -> Gain140/1, Gain156/1, Tl30/3
  Sum100/1 -> Cp31/1
  Sum95/1 -> Cp30/1

== system RC_top_ACU/Global Model RC/Local Control ==
  curr_T_liquide : Inport
  %/c : RateLimiter  RisingSlewLimit=5  FallingSlewLimit=-5  SampleTimeMode=inherited
  Display2 : Display
  "Kdta, mA/C" : Gain  Gain=0.08
  Kpi : Gain
  Kro : Gain  Gain=0.006
  "Kzd, mA/C" : Gain  Gain=0.08
  Sum29 : Sum  Inputs=+-
  Sum30 : Sum
  Ti : Integrator  InitialCondition=8000  UpperSaturationLimit=8012  LowerSaturationLimit=6012
  "Tz, C" : Constant  Value=160.00
  "pozicioner, %/mA" : Gain  Gain=6.25
  curr_T_flue : Outport
  wires:
  Ti/1 -> Sum30/2
  Kpi/1 -> Ti/1, Sum30/1
  "Tz, C"/1 -> "Kzd, mA/C"/1
  "Kzd, mA/C"/1 -> Sum29/1
  %/c/1 -> Kro/1
  "Kdta, mA/C"/1 -> Sum29/2
  curr_T_liquide/1 -> "Kdta, mA/C"/1
  "pozicioner, %/mA"/1 -> %/c/1
  Sum30/1 -> "pozicioner, %/mA"/1
  Kro/1 -> curr_T_flue/1, Display2/1
  Sum29/1 -> Kpi/1

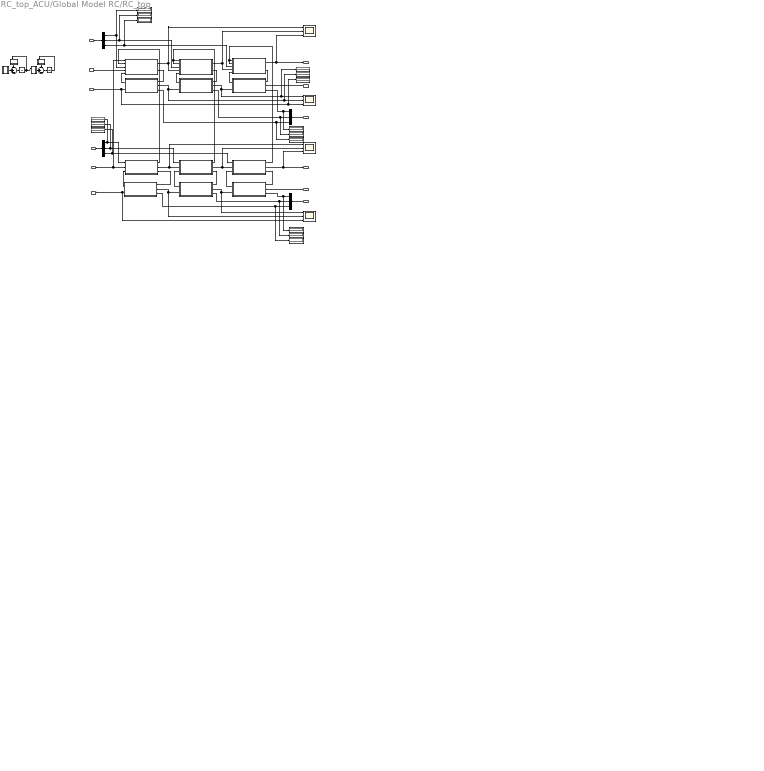
== system RC_top_ACU/Global Model RC/RC_top ==
  note: 129.39435000
  note: 126.38880000
  note: 123.38325000
  init_condition_C_steam : Inport
  init_condition_C_liquide : Inport  Port=2
  init_condition_T_steam : Inport  Port=3
  init_condition_T_liquide : Inport  Port=4
  C_steam_prev_point : Inport  Port=5
  C_liquide_prev_point : Inport  Port=6
  T_steam_prev_point : Inport  Port=7
  T_liquide_prev_point : Inport  Port=8
  C_liquide : Scope  NumInputPorts=3
  C_liquide_1 : Subsystem
  C_liquide_2 : Subsystem
  C_liquide_3 : Subsystem
  C_steam : Scope  NumInputPorts=3
  C_steam_1 : Subsystem
  C_steam_2 : Subsystem
  C_steam_3 : Subsystem
  Cp1 : Integrator  InitialCondition=0.68200000
  Cp2 : Integrator  InitialCondition=0.83400000
  Demux{1..4} (4 alike) : Demux  Outputs=3
  Display{,1..14} (15 alike) : Display
  Sum6 : Sum  Inputs=-+-
  Sum7 : Sum  Inputs=-+-
  T_liquide : Scope  NumInputPorts=3
  T_liquide_1 : Subsystem
  T_liquide_2 : Subsystem
  T_liquide_3 : Subsystem
  T_steam : Scope  NumInputPorts=3
  T_steam_1 : Subsystem
  T_steam_2 : Subsystem
  T_steam_3 : Subsystem
  k1 : Subsystem
  k2 : Subsystem
  speed1 : Subsystem
  speed6 : Subsystem
  C_steam_next_point : Outport
  C_liquide_next_point : Outport  Port=2
  T_steam_next_point : Outport  Port=3
  T_liquide_next_point : Outport  Port=4
  wires:
  T_steam_2/2(to_next_point) -> T_steam_3/2(from_prev_point), T_steam/2
  T_steam_3/2(to_next_point) -> T_steam_next_point/1, T_steam/3
  T_steam_prev_point/1 -> C_steam_1/1(from_T_prev_point), T_steam_1/2(from_prev_point)
  T_liquide_1/1(to_steam) -> T_steam_3/3(from_liquid)
  T_steam_3/3(to_liquid) -> T_liquide_1/1(from_steam)
  T_liquide_prev_point/1 -> T_liquide_1/2(from_prev_point)
  T_liquide_1/2(to_next_point) -> T_liquide_2/2(from_prev_point), T_liquide/1
  T_steam_2/3(to_liquid) -> T_liquide_2/1(from_steam)
  T_liquide_2/1(to_steam) -> T_steam_2/3(from_liquid)
  T_liquide_2/2(to_next_point) -> T_liquide_3/2(from_prev_point), T_liquide/2
  T_steam_1/3(to_liquid) -> T_liquide_3/1(from_steam)
  T_liquide_3/1(to_steam) -> T_steam_1/3(from_liquid)
  Demux4/2 -> T_liquide_2/3(init_condition_curr_point), Display10/1
  Demux4/3 -> T_liquide_3/3(init_condition_curr_point), Display11/1
  T_liquide_3/2(to_next_point) -> T_liquide/3, T_liquide_next_point/1
  C_liquide_3/1(to_steam) -> C_steam_1/5(from_liquid)
  C_steam_3/1(to_next_point) -> C_steam/3, C_steam_next_point/1
  C_steam_1/1(to_next_point) -> C_steam_2/4(from_prev_point), C_steam/1
  Demux3/3 -> C_steam_3/3(init_condition_curr_point), Display2/1
  C_steam_3/2(to_liquid) -> C_liquide_1/1(from_steam)
  C_liquide_prev_point/1 -> C_liquide_1/2(from_prev_point)
  C_liquide_2/2(to_next_point) -> C_liquide_3/2(from_prev_point), Display13/1, C_liquide/2
  C_steam_2/2(to_liquid) -> C_liquide_2/1(from_steam)
  C_liquide_1/1(to_steam) -> C_steam_3/5(from_liquid)
  C_liquide_3/2(to_next_point) -> Display14/1, C_liquide/3, C_liquide_next_point/1
  Demux1/2 -> C_liquide_2/3(init_condition_curr_point), Display4/1
  Demux1/3 -> C_liquide_3/3(init_condition_curr_point), Display5/1
  C_steam_prev_point/1 -> C_steam_1/4(from_prev_point)
  C_steam_1/2(to_liquid) -> C_liquide_3/1(from_steam)
  C_liquide_2/1(to_steam) -> C_steam_2/5(from_liquid)
  C_liquide_1/2(to_next_point) -> C_liquide_2/2(from_prev_point), Display12/1, C_liquide/1
  init_condition_T_steam/1 -> Demux2/1
  Demux2/1 -> T_steam_1/1(init_condition_curr_point), Display6/1
  Demux2/3 -> T_steam_3/1(init_condition_curr_point), Display8/1
  init_condition_T_liquide/1 -> Demux4/1
  Demux4/1 -> Display9/1, T_liquide_1/3(init_condition_curr_point)
  init_condition_C_steam/1 -> Demux3/1
  Demux3/2 -> C_steam_2/3(init_condition_curr_point), Display1/1
  init_condition_C_liquide/1 -> Demux1/1
  Demux1/1 -> C_liquide_1/3(init_condition_curr_point), Display3/1
  C_steam_2/1(to_next_point) -> C_steam/2, C_steam_3/4(from_prev_point)
  T_steam_2/1(to_concentration) -> C_steam_2/1(from_T_prev_point), C_steam_2/2(from_T_curr_point)
  T_steam_3/1(to_concentration) -> C_steam_3/1(from_T_prev_point), C_steam_3/2(from_T_curr_point)
  Demux2/2 -> T_steam_2/1(init_condition_curr_point), Display7/1
  T_steam_1/2(to_next_point) -> T_steam_2/2(from_prev_point), T_steam/1
  Demux3/1 -> Display/1, C_steam_1/3(init_condition_curr_point)
  T_steam_1/1(to_concentration) -> C_steam_1/2(from_T_curr_point)
  Cp2/1 -> k2/1(In1)
  k1/1(Out1) -> Sum6/1
  k2/1(Out1) -> Sum7/1
  speed6/1(Out1) -> Sum6/2
  ? -> speed6/1(In1)
  Sum7/1 -> Cp2/1
  speed1/1(Out1) -> Sum7/2
  Sum6/1 -> Cp1/1
  Cp1/1 -> k1/1(In1), speed1/1(In1)

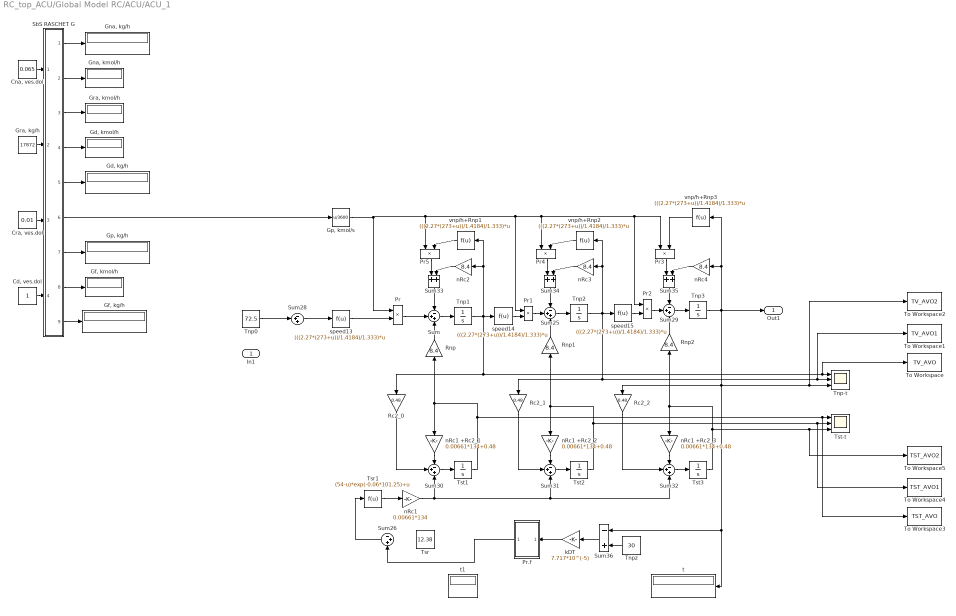
== system RC_top_ACU/Global Model RC/ACU/ACU_1  ==
  In1 : Inport
  "Cd, ves.dol" : Constant
  "Cna, ves.dol" : Constant  Value=0.065
  "Cra, ves.dol" : Constant  Value=0.01
  "Gd, kg/h" : Display
  "Gd, kmol/h" : Display
  "Gf, kg/h" : Display
  "Gf, kmol/h" : Display
  "Gna, kg/h" : Display
  "Gna, kmol/h" : Display
  "Gp, kmol/s" : Fcn  Expr=u/3600
  "Gp, kg/h" : Display
  "Gra, kg/h" : Constant  Value=17872
  "Gra, kmol/h" : Display
  Pr{,1..5} (6 alike) : Product  RndMeth=Zero
  Pr.f : Subsystem
  Rc2_0 : Gain  Gain=0.48
  Rc2_1 : Gain  Gain=0.48
  Rc2_2 : Gain  Gain=0.48
  Rnp : Gain  Gain=8.4
  Rnp1 : Gain  Gain=8.4
  Rnp2 : Gain  Gain=8.4
  SbS RASCHET G : Subsystem
  Sum{,25..26,28..32} (8 alike) : Sum  Inputs=-++
  Sum33 : Sum
  Sum34 : Sum
  Sum35 : Sum
  Sum36 : Sum  Inputs=-+
  Tnp-t : Scope  NumInputPorts=3
  Tnp0 : Constant  Value=72.5
  Tnp1 : Integrator  InitialCondition=64.99850000
  Tnp2 : Integrator  InitialCondition=57.49700000
  Tnp3 : Integrator  InitialCondition=49.99550000
  Tnpz : Constant  Value=30
  To Workspace : ToWorkspace  VariableName=TV_AVO  SaveFormat=Structure With Time  SampleTime=-1
  To Workspace1 : ToWorkspace  VariableName=TV_AVO1  SaveFormat=Structure With Time  SampleTime=-1
  To Workspace2 : ToWorkspace  VariableName=TV_AVO2  SaveFormat=Structure With Time  SampleTime=-1
  To Workspace3 : ToWorkspace  VariableName=TST_AVO  SaveFormat=Structure With Time  SampleTime=-1
  To Workspace4 : ToWorkspace  VariableName=TST_AVO1  SaveFormat=Structure With Time  SampleTime=-1
  To Workspace5 : ToWorkspace  VariableName=TST_AVO2  SaveFormat=Structure With Time  SampleTime=-1
  Tsr : Constant  Value=12.38
  Tsr1 : Fcn  Expr=(54-u)*exp(-0.06*101.25)+u
  Tst-t : Scope  NumInputPorts=3
  Tst1 : Integrator  InitialCondition=30.749212884999000
  Tst2 : Integrator  InitialCondition=26.338794670104530
  Tst3 : Integrator  InitialCondition=23.289742144317184
  kDT : Gain  Gain=7.717*10^(-5)
  nRc1 : Gain  Gain=0.00661*134
  nRc1 +Rc2_1 : Gain  Gain=0.00661*134+0.48
  nRc1 +Rc2_2 : Gain  Gain=0.00661*134+0.48
  nRc1 +Rc2_3 : Gain  Gain=0.00661*134+0.48
  nRc2 : Gain  Gain=8.4
  nRc3 : Gain  Gain=8.4
  nRc4 : Gain  Gain=8.4
  speed13 : Fcn  Expr=(((2.27*(273+u))/1.4184)/1.333)*u
  speed14 : Fcn  Expr=(((2.27*(273+u))/1.4184)/1.333)*u
  speed15 : Fcn  Expr=(((2.27*(273+u))/1.4184)/1.333)*u
  t : Display
  t1 : Display
  vnp/h+Rnp1 : Fcn  Expr=(((2.27*(273+u))/1.4184)/1.333)*u
  vnp/h+Rnp2 : Fcn  Expr=(((2.27*(273+u))/1.4184)/1.333)*u
  vnp/h+Rnp3 : Fcn  Expr=(((2.27*(273+u))/1.4184)/1.333)*u
  Out1 : Outport
  wires:
  nRc1 +Rc2_3/1 -> Sum32/1
  Tnp0/1 -> Sum28/2
  Rc2_2/1 -> Sum32/2
  nRc2/1 -> Sum33/2
  Pr2/1 -> Sum29/2
  "Gra, kg/h"/1 -> SbS RASCHET G/2(In2)
  Sum31/1 -> Tst2/1
  Pr5/1 -> Sum33/1
  Pr1/1 -> Sum25/2
  nRc1 +Rc2_2/1 -> Sum31/1
  Rnp1/1 -> Sum25/3
  speed14/1 -> Pr1/2
  vnp/h+Rnp3/1 -> Pr3/2
  Rnp/1 -> Sum/3
  nRc3/1 -> Sum34/2
  Rnp2/1 -> Sum29/3
  Sum25/1 -> Tnp2/1
  SbS RASCHET G/5(Out5) -> "Gd, kg/h"/1
  Tnp2/1 -> speed15/1, Rc2_1/1, To Workspace1/1, Tnp-t/2, vnp/h+Rnp2/1, nRc3/1
  Sum/1 -> Tnp1/1
  SbS RASCHET G/9(Out9) -> "Gf, kg/h"/1
  kDT/1 -> Pr.f/1(In1)
  "Cra, ves.dol"/1 -> SbS RASCHET G/3(In3)
  Pr.f/1(Out1) -> Sum26/3
  Sum28/1 -> speed13/1
  SbS RASCHET G/3(Out3) -> "Gra, kmol/h"/1
  speed13/1 -> Pr/2
  SbS RASCHET G/1(Out1) -> "Gna, kg/h"/1
  nRc1 +Rc2_1/1 -> Sum30/1
  Sum32/1 -> Tst3/1
  Tnp1/1 -> speed14/1, Rc2_0/1, To Workspace/1, Tnp-t/1, vnp/h+Rnp1/1, nRc2/1
  "Cd, ves.dol"/1 -> SbS RASCHET G/4(In4)
  Sum36/1 -> kDT/1
  Tst2/1 -> nRc1 +Rc2_2/1, Rnp1/1, To Workspace4/1, Tst-t/2
  Pr4/1 -> Sum34/1
  Tsr1/1 -> nRc1/1
  Pr/1 -> Sum/2
  Tnp3/1 -> vnp/h+Rnp3/1, nRc4/1, Out1/1, To Workspace2/1, Tnp-t/3, t/1, Sum36/1, Rc2_2/1
  Tst1/1 -> nRc1 +Rc2_1/1, Rnp/1, Tst-t/1, To Workspace3/1
  Pr3/1 -> Sum35/1
  speed15/1 -> Pr2/2
  SbS RASCHET G/6(Out6) -> "Gp, kmol/s"/1
  vnp/h+Rnp2/1 -> Pr4/2
  vnp/h+Rnp1/1 -> Pr5/2
  SbS RASCHET G/2(Out2) -> "Gna, kmol/h"/1
  SbS RASCHET G/8(Out8) -> "Gf, kmol/h"/1
  "Gp, kmol/s"/1 -> Pr/1, Pr5/1, Pr1/1, Pr4/1, Pr2/1, Pr3/1
  nRc1/1 -> Sum30/3, Sum31/3, Sum32/3
  Sum26/1 -> Tsr1/1
  Sum33/1 -> Sum/1
  Tnpz/1 -> Sum36/2
  SbS RASCHET G/7(Out7) -> "Gp, kg/h"/1
  SbS RASCHET G/4(Out4) -> "Gd, kmol/h"/1
  Rc2_1/1 -> Sum31/2
  Sum29/1 -> Tnp3/1
  "Cna, ves.dol"/1 -> SbS RASCHET G/1(In1)
  Sum30/1 -> Tst1/1
  Rc2_0/1 -> Sum30/2
  Sum34/1 -> Sum25/1
  nRc4/1 -> Sum35/2
  Sum35/1 -> Sum29/1
  Tst3/1 -> nRc1 +Rc2_3/1, Rnp2/1, To Workspace5/1, Tst-t/3

== system RC_top_ACU/Global Model RC/ACU/C_liquide_1 ==
  from_steam : Inport
  from_prev_point : Inport  Port=2
  init_condition_curr_point : Inport  Port=3
  Gain18 : Gain  Gain=0.000004000
  Gain19 : Gain  Gain=0.003/1.375
  Gain22 : Gain  Gain=0.003/1.375-(0.000004000)*10^(-9)
  Sum2 : Sum  Inputs=-+-
  Tl1 : Integrator  InitialConditionSource=external  InitialCondition=124.3766
  to_steam : Outport
  to_next_point : Outport  Port=2
  wires:
  from_steam/1 -> Gain18/1
  from_prev_point/1 -> Gain19/1
  Gain19/1 -> Sum2/2
  Sum2/1 -> Tl1/1
  Gain18/1 -> Sum2/1
  init_condition_curr_point/1 -> Tl1/2
  Gain22/1 -> Sum2/3
  Tl1/1 -> Gain22/1, to_steam/1, to_next_point/1

== system RC_top_ACU/Global Model RC/ACU/C_liquide_2 ==
  from_steam : Inport
  from_prev_point : Inport  Port=2
  init_condition_curr_point : Inport  Port=3
  Gain18 : Gain  Gain=0.000004000
  Gain19 : Gain  Gain=0.003/1.375
  Gain22 : Gain  Gain=0.003/1.375-(0.000004000)*10^(-9)
  Sum2 : Sum  Inputs=-+-
  Tl1 : Integrator  InitialConditionSource=external  InitialCondition=124.3766
  to_steam : Outport
  to_next_point : Outport  Port=2
  wires:
  from_steam/1 -> Gain18/1
  from_prev_point/1 -> Gain19/1
  Gain19/1 -> Sum2/2
  Sum2/1 -> Tl1/1
  Gain18/1 -> Sum2/1
  init_condition_curr_point/1 -> Tl1/2
  Gain22/1 -> Sum2/3
  Tl1/1 -> Gain22/1, to_steam/1, to_next_point/1

== system RC_top_ACU/Global Model RC/ACU/C_liquide_3 ==
  from_steam : Inport
  from_prev_point : Inport  Port=2
  init_condition_curr_point : Inport  Port=3
  Gain18 : Gain  Gain=0.000004000
  Gain19 : Gain  Gain=0.003/1.375
  Gain22 : Gain  Gain=0.003/1.375-(0.000004000)*10^(-9)
  Sum2 : Sum  Inputs=-+-
  Tl1 : Integrator  InitialConditionSource=external  InitialCondition=124.3766
  to_steam : Outport
  to_next_point : Outport  Port=2
  wires:
  from_steam/1 -> Gain18/1
  from_prev_point/1 -> Gain19/1
  Gain19/1 -> Sum2/2
  Sum2/1 -> Tl1/1
  Gain18/1 -> Sum2/1
  init_condition_curr_point/1 -> Tl1/2
  Gain22/1 -> Sum2/3
  Tl1/1 -> Gain22/1, to_steam/1, to_next_point/1

== system RC_top_ACU/Global Model RC/ACU/C_liquide_4 ==
  from_steam : Inport
  from_prev_point : Inport  Port=2
  init_condition_curr_point : Inport  Port=3
  Gain18 : Gain  Gain=0.000004000
  Gain19 : Gain  Gain=0.003/1.375
  Gain22 : Gain  Gain=0.003/1.375-(0.000004000)*10^(-9)
  Sum2 : Sum  Inputs=-+-
  Tl1 : Integrator  InitialConditionSource=external  InitialCondition=124.3766
  to_steam : Outport
  to_next_point : Outport  Port=2
  wires:
  from_steam/1 -> Gain18/1
  from_prev_point/1 -> Gain19/1
  Gain19/1 -> Sum2/2
  Sum2/1 -> Tl1/1
  Gain18/1 -> Sum2/1
  init_condition_curr_point/1 -> Tl1/2
  Gain22/1 -> Sum2/3
  Tl1/1 -> Gain22/1, to_steam/1, to_next_point/1

== system RC_top_ACU/Global Model RC/ACU/C_steam ==
  point_1 : Inport
  point_3 : Inport  Port=2
  point_2 : Inport  Port=3
  point_4 : Inport  Port=4
  Gain : Gain  Gain=1/4
  Sum37 : Sum  Inputs=++++
  to_side : Outport
  wires:
  point_2/1 -> Sum37/2
  point_1/1 -> Sum37/1
  point_3/1 -> Sum37/3
  point_4/1 -> Sum37/4
  Sum37/1 -> Gain/1
  Gain/1 -> to_side/1

== system RC_top_ACU/Global Model RC/ACU/C_steam_1 ==
  from_T_prev_point : Inport
  from_T_curr_point : Inport  Port=2
  init_condition_curr_point : Inport  Port=3
  EVAP_params : Inport  Port=4
  from_prev_point : Inport  Port=5
  from_liquid : Inport  Port=6
  C_steam : Integrator  InitialConditionSource=external  InitialCondition=156.9966
  Gain29 : Gain  Gain=0.0000216487318*10^(-9)
  Sum3 : Sum  Inputs=-+-
  k1 : Subsystem
  speed : Subsystem
  to_next_point : Outport
  to_liquid : Outport  Port=2
  wires:
  init_condition_curr_point/1 -> C_steam/2
  speed/1(Out1) -> Sum3/2
  Gain29/1 -> Sum3/3
  Sum3/1 -> C_steam/1
  from_liquid/1 -> Gain29/1
  k1/1(Out1) -> Sum3/1
  C_steam/1 -> k1/2(In2), to_next_point/1, to_liquid/1
  from_T_curr_point/1 -> k1/1(In1)
  EVAP_params/1 -> k1/3(EVAP_params1), speed/3(EVAP_params)
  from_prev_point/1 -> speed/1(In1)
  from_T_prev_point/1 -> speed/2(In2)

== system RC_top_ACU/Global Model RC/ACU/C_steam_2 ==
  from_T_prev_point : Inport
  from_T_curr_point : Inport  Port=2
  init_condition_curr_point : Inport  Port=3
  EVAP_params : Inport  Port=4
  from_prev_point : Inport  Port=5
  from_liquid : Inport  Port=6
  C_steam : Integrator  InitialConditionSource=external  InitialCondition=156.9966
  Gain29 : Gain  Gain=0.0000216487318*10^(-9)
  Sum3 : Sum  Inputs=-+-
  k1 : Subsystem
  speed : Subsystem
  to_next_point : Outport
  to_liquid : Outport  Port=2
  wires:
  init_condition_curr_point/1 -> C_steam/2
  speed/1(Out1) -> Sum3/2
  Gain29/1 -> Sum3/3
  Sum3/1 -> C_steam/1
  from_liquid/1 -> Gain29/1
  k1/1(Out1) -> Sum3/1
  C_steam/1 -> k1/2(In2), to_next_point/1, to_liquid/1
  from_T_curr_point/1 -> k1/1(In1)
  EVAP_params/1 -> k1/3(EVAP_params1), speed/3(EVAP_params)
  from_prev_point/1 -> speed/1(In1)
  from_T_prev_point/1 -> speed/2(In2)

== system RC_top_ACU/Global Model RC/ACU/C_steam_3 ==
  from_T_prev_point : Inport
  from_T_curr_point : Inport  Port=2
  init_condition_curr_point : Inport  Port=3
  EVAP_params : Inport  Port=4
  from_prev_point : Inport  Port=5
  from_liquid : Inport  Port=6
  C_steam : Integrator  InitialConditionSource=external  InitialCondition=156.9966
  Gain29 : Gain  Gain=0.0000216487318*10^(-9)
  Sum3 : Sum  Inputs=-+-
  k1 : Subsystem
  speed : Subsystem
  to_next_point : Outport
  to_liquid : Outport  Port=2
  wires:
  init_condition_curr_point/1 -> C_steam/2
  speed/1(Out1) -> Sum3/2
  Gain29/1 -> Sum3/3
  Sum3/1 -> C_steam/1
  from_liquid/1 -> Gain29/1
  k1/1(Out1) -> Sum3/1
  C_steam/1 -> k1/2(In2), to_next_point/1, to_liquid/1
  from_T_curr_point/1 -> k1/1(In1)
  EVAP_params/1 -> k1/3(EVAP_params1), speed/3(EVAP_params)
  from_prev_point/1 -> speed/1(In1)
  from_T_prev_point/1 -> speed/2(In2)
